simulink model "ER_Simulink"  (R2016b)
settings: Solver=VariableStepAuto  StartTime=0.01  StopTime=10.0  RelTol=1e-3  EnableMultiTasking=on
undefined symbols (not defined in the file or in its folder): sigbuilder_block
settings Model: Creator=Administrator  LastModifiedBy=maelula
settings DataIOCC: LimitDataPoints=on  SaveFormat=Array
settings OptimizationCC: LifeSpan=inf
settings DebuggingCC: SolverPrmCheckMsg=warning  SFUnexpectedBacktrackingDiag=warning  SFNoUnconditionalDefaultTransitionDiag=warning  SFExecutionAtInitializationDiag=none
settings HardwareCC: ProdBitPerPointer=32  ProdBitPerSizeT=32  ProdBitPerPtrDiffT=32  ProdLargestAtomicFloat=None  ProdIntDivRoundTo=Undefined  ProdEndianess=Unspecified  ProdWordSize=32  ProdHWDeviceType=32-bit Generic
settings ModelReferenceCC: PropagateSignalLabelsOutOfModel=off
settings GRTTargetCC: TargetLangStandard=C89/C90 (ANSI)  GeneratePreprocessorConditionals=Disable all
settings ConfigComp: CovMetricSettings=dw  CovHtmlReporting=on  CovSaveCumulativeToWorkspaceVar=on  CovSaveSingleToWorkspaceVar=on  CovExternalEMLEnable=off  CovSFcnEnable=off

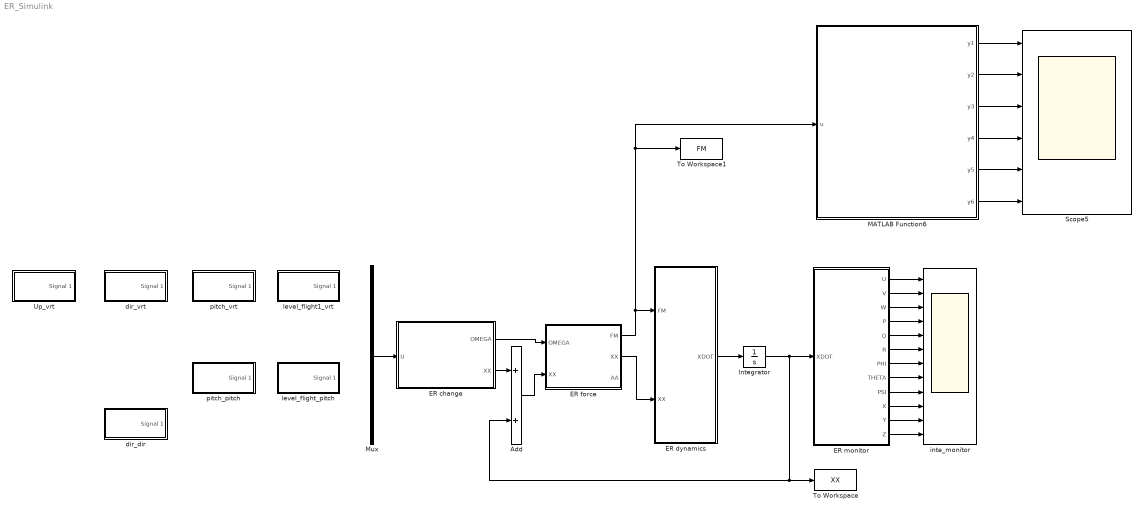
== system ER_Simulink ==
  Add : Sum
  "ER change " : MATLAB Function  TreatAsAtomicUnit=on
  "ER dynamics " : MATLAB Function  TreatAsAtomicUnit=on
  ER force : MATLAB Function  TreatAsAtomicUnit=on
  ER monitor : MATLAB Function  TreatAsAtomicUnit=on
  Integrator : Integrator
  MATLAB Function6 : MATLAB Function  TreatAsAtomicUnit=on
  Mux : Mux
  Scope5 : Scope  NumInputPorts=6
  To Workspace : ToWorkspace  VariableName=XX  SampleTime=-1
  To Workspace1 : ToWorkspace  VariableName=FM  SampleTime=-1
  Up_vrt : Subsystem  Tag=STV Subsys  LoadFcn=sigbuilder_block('load');  StartFcn=sigbuilder_block('start');  StopFcn=sigbuilder_block('stop');  ClipboardFcn=sigbuilder_block('clipboard');  mask(Sigbuilder block){tuvar=[0:10]}
      mask help: Simulink:masks:SigbuilderBlock_MD
      mask init:
      | if ~strcmp(get_param(bdroot(gcbh),'SimulationStatus'),'stopped') tuvar = sigbuilder_block('maskInit'); end
      settings: CopyFcn=sigbuilder_block('copy');  DeleteFcn=sigbuilder_block('delete');  ModelCloseFcn=sigbuilder_block('modelClose');  PreSaveFcn=sigbuilder_block('preSave');  PauseFcn=sigbuilder_block('pause');  ContinueFcn=sigbuilder_block('continue');  NameChangeFcn=sigbuilder_block('namechange');  OpenFcn=sigbuilder_block('open',[327 194 749 530 ]);  CloseFcn=sigbuilder_block('close');
      mask Display: plot(0, 0, 100, 100,[2, 2, 32, 32, 2], [68, 8, 8, 68, 68],[32, 2], [38, 38], [32, 19, 2],[53, 60, 44], [32, 17, 17, 2],[16, 16, 31, 31]);txt = getActiveGroup(gcbh);text(2, 100, txt,'verticalAlignment', 'top');
  dir_dir : Subsystem  Tag=STV Subsys  LoadFcn=sigbuilder_block('load');  StartFcn=sigbuilder_block('start');  StopFcn=sigbuilder_block('stop');  ClipboardFcn=sigbuilder_block('clipboard');  mask(Sigbuilder block){tuvar=[0:10]}
      mask help: Simulink:masks:SigbuilderBlock_MD
      mask init:
      | if ~strcmp(get_param(bdroot(gcbh),'SimulationStatus'),'stopped') tuvar = sigbuilder_block('maskInit'); end
      settings: CopyFcn=sigbuilder_block('copy');  DeleteFcn=sigbuilder_block('delete');  ModelCloseFcn=sigbuilder_block('modelClose');  PreSaveFcn=sigbuilder_block('preSave');  PauseFcn=sigbuilder_block('pause');  ContinueFcn=sigbuilder_block('continue');  NameChangeFcn=sigbuilder_block('namechange');  OpenFcn=sigbuilder_block('open',[304 160 891 552 ]);  CloseFcn=sigbuilder_block('close');
      mask Display: plot(0, 0, 100, 100,[2, 2, 32, 32, 2], [68, 8, 8, 68, 68],[32, 2], [38, 38], [32, 19, 2],[53, 60, 44], [32, 17, 17, 2],[16, 16, 31, 31]);txt = getActiveGroup(gcbh);text(2, 100, txt,'verticalAlignment', 'top');
  dir_vrt : Subsystem  Tag=STV Subsys  LoadFcn=sigbuilder_block('load');  StartFcn=sigbuilder_block('start');  StopFcn=sigbuilder_block('stop');  ClipboardFcn=sigbuilder_block('clipboard');  mask(Sigbuilder block){tuvar=[0:10]}
      mask help: Simulink:masks:SigbuilderBlock_MD
      mask init:
      | if ~strcmp(get_param(bdroot(gcbh),'SimulationStatus'),'stopped') tuvar = sigbuilder_block('maskInit'); end
      settings: CopyFcn=sigbuilder_block('copy');  DeleteFcn=sigbuilder_block('delete');  ModelCloseFcn=sigbuilder_block('modelClose');  PreSaveFcn=sigbuilder_block('preSave');  PauseFcn=sigbuilder_block('pause');  ContinueFcn=sigbuilder_block('continue');  NameChangeFcn=sigbuilder_block('namechange');  OpenFcn=sigbuilder_block('open',[232 176 799 559 ]);  CloseFcn=sigbuilder_block('close');
      mask Display: plot(0, 0, 100, 100,[2, 2, 32, 32, 2], [68, 8, 8, 68, 68],[32, 2], [38, 38], [32, 19, 2],[53, 60, 44], [32, 17, 17, 2],[16, 16, 31, 31]);txt = getActiveGroup(gcbh);text(2, 100, txt,'verticalAlignment', 'top');
  inte_monitor : Scope  NumInputPorts=12
  "level_flight1_vrt " : Subsystem  Tag=STV Subsys  LoadFcn=sigbuilder_block('load');  StartFcn=sigbuilder_block('start');  StopFcn=sigbuilder_block('stop');  ClipboardFcn=sigbuilder_block('clipboard');  mask(Sigbuilder block){tuvar=[0:10]}
      mask help: Simulink:masks:SigbuilderBlock_MD
      mask init:
      | if ~strcmp(get_param(bdroot(gcbh),'SimulationStatus'),'stopped') tuvar = sigbuilder_block('maskInit'); end
      settings: CopyFcn=sigbuilder_block('copy');  DeleteFcn=sigbuilder_block('delete');  ModelCloseFcn=sigbuilder_block('modelClose');  PreSaveFcn=sigbuilder_block('preSave');  PauseFcn=sigbuilder_block('pause');  ContinueFcn=sigbuilder_block('continue');  NameChangeFcn=sigbuilder_block('namechange');  OpenFcn=sigbuilder_block('open',[470 231 709 500 ]);  CloseFcn=sigbuilder_block('close');
      mask Display: plot(0, 0, 100, 100,[2, 2, 32, 32, 2], [68, 8, 8, 68, 68],[32, 2], [38, 38], [32, 19, 2],[53, 60, 44], [32, 17, 17, 2],[16, 16, 31, 31]);txt = getActiveGroup(gcbh);text(2, 100, txt,'verticalAlignment', 'top');
  level_flight_pitch : Subsystem  Tag=STV Subsys  LoadFcn=sigbuilder_block('load');  StartFcn=sigbuilder_block('start');  StopFcn=sigbuilder_block('stop');  ClipboardFcn=sigbuilder_block('clipboard');  mask(Sigbuilder block){tuvar=[0:10]}
      mask help: Simulink:masks:SigbuilderBlock_MD
      mask init:
      | if ~strcmp(get_param(bdroot(gcbh),'SimulationStatus'),'stopped') tuvar = sigbuilder_block('maskInit'); end
      settings: CopyFcn=sigbuilder_block('copy');  DeleteFcn=sigbuilder_block('delete');  ModelCloseFcn=sigbuilder_block('modelClose');  PreSaveFcn=sigbuilder_block('preSave');  PauseFcn=sigbuilder_block('pause');  ContinueFcn=sigbuilder_block('continue');  NameChangeFcn=sigbuilder_block('namechange');  OpenFcn=sigbuilder_block('open',[139 266 709 484 ]);  CloseFcn=sigbuilder_block('close');
      mask Display: plot(0, 0, 100, 100,[2, 2, 32, 32, 2], [68, 8, 8, 68, 68],[32, 2], [38, 38], [32, 19, 2],[53, 60, 44], [32, 17, 17, 2],[16, 16, 31, 31]);txt = getActiveGroup(gcbh);text(2, 100, txt,'verticalAlignment', 'top');
  pitch_pitch : Subsystem  Tag=STV Subsys  LoadFcn=sigbuilder_block('load');  StartFcn=sigbuilder_block('start');  StopFcn=sigbuilder_block('stop');  ClipboardFcn=sigbuilder_block('clipboard');  mask(Sigbuilder block){tuvar=[0:10]}
      mask help: Simulink:masks:SigbuilderBlock_MD
      mask init:
      | if ~strcmp(get_param(bdroot(gcbh),'SimulationStatus'),'stopped') tuvar = sigbuilder_block('maskInit'); end
      settings: CopyFcn=sigbuilder_block('copy');  DeleteFcn=sigbuilder_block('delete');  ModelCloseFcn=sigbuilder_block('modelClose');  PreSaveFcn=sigbuilder_block('preSave');  PauseFcn=sigbuilder_block('pause');  ContinueFcn=sigbuilder_block('continue');  NameChangeFcn=sigbuilder_block('namechange');  OpenFcn=sigbuilder_block('open',[139 266 709 484 ]);  CloseFcn=sigbuilder_block('close');
      mask Display: plot(0, 0, 100, 100,[2, 2, 32, 32, 2], [68, 8, 8, 68, 68],[32, 2], [38, 38], [32, 19, 2],[53, 60, 44], [32, 17, 17, 2],[16, 16, 31, 31]);txt = getActiveGroup(gcbh);text(2, 100, txt,'verticalAlignment', 'top');
  pitch_vrt : Subsystem  Tag=STV Subsys  LoadFcn=sigbuilder_block('load');  StartFcn=sigbuilder_block('start');  StopFcn=sigbuilder_block('stop');  ClipboardFcn=sigbuilder_block('clipboard');  mask(Sigbuilder block){tuvar=[0:10]}
      mask help: Simulink:masks:SigbuilderBlock_MD
      mask init:
      | if ~strcmp(get_param(bdroot(gcbh),'SimulationStatus'),'stopped') tuvar = sigbuilder_block('maskInit'); end
      settings: CopyFcn=sigbuilder_block('copy');  DeleteFcn=sigbuilder_block('delete');  ModelCloseFcn=sigbuilder_block('modelClose');  PreSaveFcn=sigbuilder_block('preSave');  PauseFcn=sigbuilder_block('pause');  ContinueFcn=sigbuilder_block('continue');  NameChangeFcn=sigbuilder_block('namechange');  OpenFcn=sigbuilder_block('open',[232 176 799 559 ]);  CloseFcn=sigbuilder_block('close');
      mask Display: plot(0, 0, 100, 100,[2, 2, 32, 32, 2], [68, 8, 8, 68, 68],[32, 2], [38, 38], [32, 19, 2],[53, 60, 44], [32, 17, 17, 2],[16, 16, 31, 31]);txt = getActiveGroup(gcbh);text(2, 100, txt,'verticalAlignment', 'top');
  wires:
  "ER change "/1(OMEGA) -> ER force/1(OMEGA)
  Mux/1 -> "ER change "/1(U)
  ER monitor/2(V) -> inte_monitor/2
  ER monitor/4(P) -> inte_monitor/4
  ER monitor/5(Q) -> inte_monitor/5
  ER monitor/6(R) -> inte_monitor/6
  ER monitor/8(THETA) -> inte_monitor/8
  ER monitor/11(Y) -> inte_monitor/11
  ER monitor/7(PHI) -> inte_monitor/7
  ER monitor/9(PSI) -> inte_monitor/9
  ER monitor/10(X) -> inte_monitor/10
  "ER dynamics "/1(XDOT) -> Integrator/1
  Add/1 -> ER force/2("XX ")
  ER force/2(XX) -> "ER dynamics "/2(XX)
  MATLAB Function6/1(y1) -> Scope5/1
  MATLAB Function6/2(y2) -> Scope5/2
  MATLAB Function6/4(y4) -> Scope5/4
  MATLAB Function6/5(y5) -> Scope5/5
  MATLAB Function6/6(y6) -> Scope5/6
  ER force/1(FM) -> "ER dynamics "/1(FM), To Workspace1/1, MATLAB Function6/1(u)
  Integrator/1 -> ER monitor/1(XDOT), To Workspace/1, Add/2
  "ER change "/2(XX) -> Add/1
  ER monitor/12(Z) -> inte_monitor/12
  ER monitor/3(W) -> inte_monitor/3
  MATLAB Function6/3(y3) -> Scope5/3
  ER monitor/1(U) -> inte_monitor/1

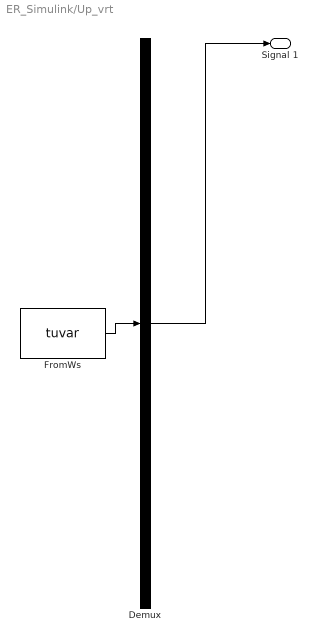
== system ER_Simulink/Up_vrt ==
  Demux : Demux  Tag=STV Demux  Outputs=1
  FromWs : FromWorkspace  Tag=STV FromWs  VariableName=tuvar  SampleTime=0
      SigBuilderData=|
      | common.afterFinalStr = 'Extrapolate'
      | common.sampleTime = 0
      | dataSet.timeRange = [0 10]
      | dataSet.name = 'Group 1'
      | sbobj.Groups.Name = 'Group 1'
      | sbobj.Groups.Signals.Name = 'Signal 1'
      | sbobj.Groups.Signals.XData = [0 3 5 10]
      | sbobj.Groups.Signals.YData = [200 200 167.1876 167.1876]
  Signal 1 : Outport  Tag=STV Outport
  wires:
  Demux/1 -> Signal 1/1
  FromWs/1 -> Demux/1

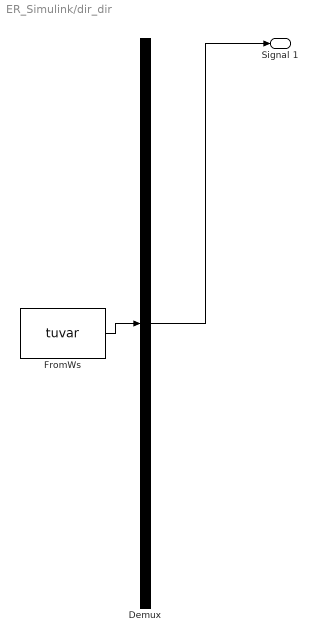
== system ER_Simulink/dir_dir ==
  Demux : Demux  Tag=STV Demux  Outputs=1
  FromWs : FromWorkspace  Tag=STV FromWs  VariableName=tuvar  SampleTime=0
      SigBuilderData=|
      | common.afterFinalStr = 'Extrapolate'
      | common.sampleTime = 0
      | dataSet.timeRange = [0 10]
      | dataSet.name = 'Group 1'
      | sbobj.Groups.Name = 'Group 1'
      | sbobj.Groups.Signals.Name = 'Signal 1'
      | sbobj.Groups.Signals.XData = [0 4 4 4.4 4.4 10]
      | sbobj.Groups.Signals.YData = [0 0 177.97 177.97 0 0]
  Signal 1 : Outport  Tag=STV Outport
  wires:
  Demux/1 -> Signal 1/1
  FromWs/1 -> Demux/1

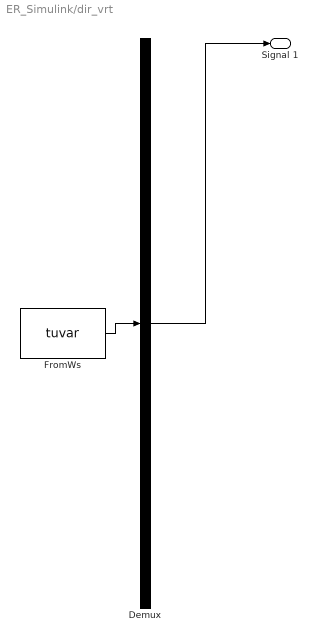
== system ER_Simulink/dir_vrt ==
  Demux : Demux  Tag=STV Demux  Outputs=1
  FromWs : FromWorkspace  Tag=STV FromWs  VariableName=tuvar  SampleTime=0
      SigBuilderData=|
      | common.afterFinalStr = 'Extrapolate'
      | common.sampleTime = 0
      | dataSet.timeRange = [0 10]
      | dataSet.name = 'Group 1'
      | sbobj.Groups.Name = 'Group 1'
      | sbobj.Groups.Signals.Name = 'Signal 1'
      | sbobj.Groups.Signals.XData = [0 1 2 5 7 10]
      | sbobj.Groups.Signals.YData = [200 200 167.188 167.188 167.1876 167.1876]
  Signal 1 : Outport  Tag=STV Outport
  wires:
  Demux/1 -> Signal 1/1
  FromWs/1 -> Demux/1

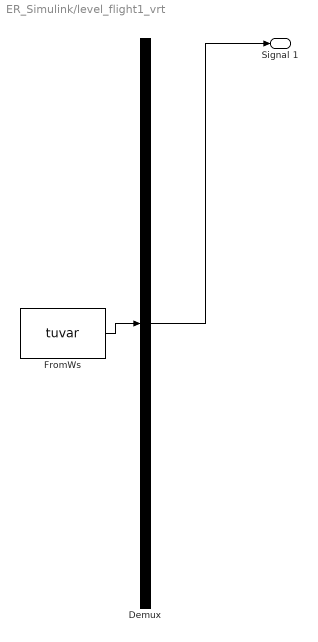
== system ER_Simulink/level_flight1_vrt  ==
  Demux : Demux  Tag=STV Demux  Outputs=1
  FromWs : FromWorkspace  Tag=STV FromWs  VariableName=tuvar  SampleTime=0
      SigBuilderData=|
      | common.afterFinalStr = 'Extrapolate'
      | common.sampleTime = 0
      | dataSet.timeRange = [0 10]
      | dataSet.name = 'Group 1'
      | sbobj.Groups.Name = 'Group 1'
      | sbobj.Groups.Signals.Name = 'Signal 1'
      | sbobj.Groups.Signals.XData = [0 1 4 6 6 10]
      | sbobj.Groups.Signals.YData = [200 200 167.1876 167.1876 198.8207 198.8207]
  Signal 1 : Outport  Tag=STV Outport
  wires:
  Demux/1 -> Signal 1/1
  FromWs/1 -> Demux/1

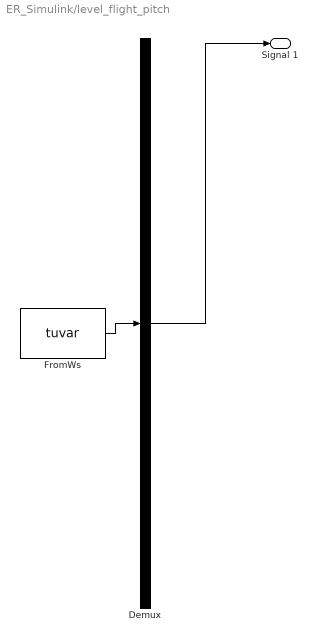
== system ER_Simulink/level_flight_pitch ==
  Demux : Demux  Tag=STV Demux  Outputs=1
  FromWs : FromWorkspace  Tag=STV FromWs  VariableName=tuvar  SampleTime=0
      SigBuilderData=|
      | common.afterFinalStr = 'Extrapolate'
      | common.sampleTime = 0
      | dataSet.timeRange = [0 10]
      | dataSet.name = 'Group 1'
      | sbobj.Groups.Name = 'Group 1'
      | sbobj.Groups.Signals.Name = 'Signal 1'
      | sbobj.Groups.Signals.XData = [0 4 4 4.4 4.4 10]
      | sbobj.Groups.Signals.YData = [0 0 62.895 62.895 0 0]
  Signal 1 : Outport  Tag=STV Outport
  wires:
  Demux/1 -> Signal 1/1
  FromWs/1 -> Demux/1

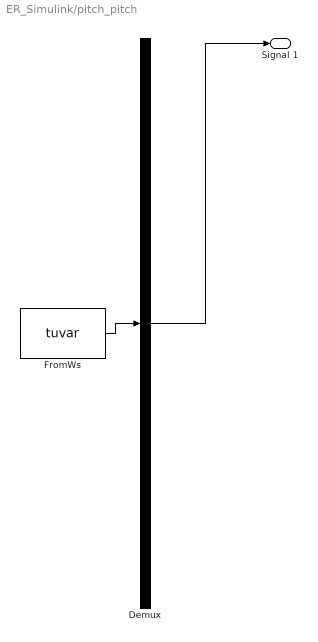
== system ER_Simulink/pitch_pitch ==
  Demux : Demux  Tag=STV Demux  Outputs=1
  FromWs : FromWorkspace  Tag=STV FromWs  VariableName=tuvar  SampleTime=0
      SigBuilderData=|
      | common.afterFinalStr = 'Extrapolate'
      | common.sampleTime = 0
      | dataSet.timeRange = [0 10]
      | dataSet.name = 'Group 1'
      | sbobj.Groups.Name = 'Group 1'
      | sbobj.Groups.Signals.Name = 'Signal 1'
      | sbobj.Groups.Signals.XData = [0 8.6 8.6 9 9 10]
      | sbobj.Groups.Signals.YData = [0 0 62.895 62.895 0 0]
  Signal 1 : Outport  Tag=STV Outport
  wires:
  Demux/1 -> Signal 1/1
  FromWs/1 -> Demux/1

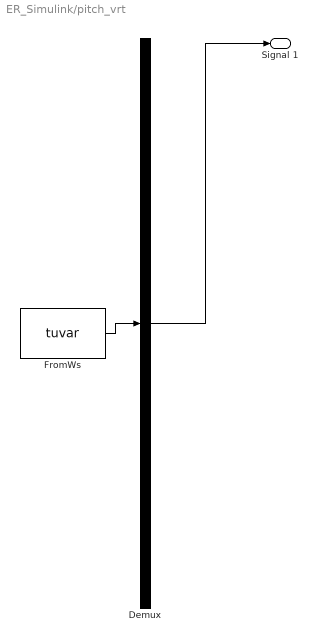
== system ER_Simulink/pitch_vrt ==
  Demux : Demux  Tag=STV Demux  Outputs=1
  FromWs : FromWorkspace  Tag=STV FromWs  VariableName=tuvar  SampleTime=0
      SigBuilderData=|
      | common.afterFinalStr = 'Extrapolate'
      | common.sampleTime = 0
      | dataSet.timeRange = [0 10]
      | dataSet.name = 'Group 1'
      | sbobj.Groups.Name = 'Group 1'
      | sbobj.Groups.Signals.Name = 'Signal 1'
      | sbobj.Groups.Signals.XData = [0 5 7 10]
      | sbobj.Groups.Signals.YData = [200 200 167.188 167.1876]
  Signal 1 : Outport  Tag=STV Outport
  wires:
  Demux/1 -> Signal 1/1
  FromWs/1 -> Demux/1

== matlab function ER_Simulink/ER change  ==
  data: U input; OMEGA output; XX output
function [OMEGA,XX]  =change(U)

%%%%%%%%%%%%%%%%%%%%%%%%%%%%%%%%%%%%%%%%%%%%%%%%
%%%%输入4个转速操纵量
Rvrt = U(1);
Rroll = U(2);
Rpitch = U(3);
Rdir = U(4);

a1=Rvrt*Rvrt;
a2=Rroll*Rroll;
a3=Rpitch*Rpitch;
a4=Rdir*Rdir;

%%%%%%%%%%%%%%%%%%%%%%%%%%%%%%%%%%%%%%%%%%%%%%%%
%%%%将转速操纵量转化为每个螺旋桨的转速
R1=a1+a2+a3-a4;
R2=a1-a2+a3+a4;
R3=a1-a2-a3-a4;
R4=a1+a2-a3+a4;
R5=a1+a2+a3+a4;
R6=a1-a2+a3-a4;
R7=a1-a2-a3+a4;
R8=a1+a2-a3-a4;


OMEGA = [R1;R2;R3;R4;R5;R6;R7;R8];

%%%%%%%%%%%%%%%%%%%%%%%%%%%%%%%%%%%%%%%%%%%%%%%%
%%%%赋予运动学量初值
XX = [0;0;0;0;0;0;0;0;0;0;0;0];

== matlab function ER_Simulink/ER dynamics  ==
  data: FM input; XX input; XDOT output
function XDOT =dynamics(FM,XX)

U = XX(1);
V = XX(2);
W = XX(3);
P = XX(4);
Q = XX(5);
R = XX(6);
PHI = XX(7);
THETA = XX(8);
PSI = XX(9);

FX = FM(1);
FY = FM(2);
FZ = FM(3);
MX = FM(4);
MY = FM(5);
MZ = FM(6);

m = 1.6;

IX = 0.0081;
IY = 0.0081;
IZ = 0.00142;

IZX = 0;

L = MX;
M = MY;
N = MZ;

%%%%%%%%%%%%%%%%%%%%%%%%%%%%%%%%%%%%%%%%%%%%%%%%
%%%%运动学方程解算
Ut = V*R-W*Q+FX/m;
Vt = -U*R+W*P+FY/m;
Wt = U*Q-V*P+FZ/m;

Pt = 1/(IX*IZ-IZX^2)*(IZ*L+IZX*N+IZX*(IX-IY+IZ)*P*Q+(IY*IZ-IZX^2-IZ^2)*Q*R);
Qt = 1/(IY)*(M-(IX-IZ)*P*R-IZX*(P^2-R^2));
Rt = 1/(IX*IZ-IZX^2)*(IZX*L+IX*N+(IX^2-IX*IY+IZX^2)*P*Q-IZX*(IX-IY-IZ)*Q*R);

PHIt = P+tan(THETA)*(Q*sin(PHI)+R*cos(PHI));
THETAt = Q*cos(PHI)-R*sin(PHI);
PSIt = 1/cos(PHI)*(Q*sin(PHI)+R*cos(PHI));

Xt = U*cos(THETA)*cos(PSI)+V*(sin(THETA)*sin(PHI)*cos(PSI)-cos(PHI)*sin(PSI))+W*(sin(THETA)*cos(PHI)*cos(PSI)+sin(PHI)*sin(PSI));
Yt = U*cos(THETA)*sin(PSI)+V*(sin(THETA)*sin(PHI)*sin(PSI)+cos(PHI)*cos(PSI))+W*(sin(THETA)*cos(PHI)*sin(PSI)-sin(PHI)*cos(PSI));
Zt = -U*sin(THETA)+V*sin(PHI)*cos(THETA)+W*cos(PHI)*cos(THETA);

XDOT = [Ut;Vt;Wt;Pt;Qt;Rt;PHIt;THETAt;PSIt;Xt;Yt;Zt];

== matlab function ER_Simulink/ER monitor ==
  data: XDOT input; U output; V output; W output; P output; Q output; R output; PHI output; THETA output; PSI output; X output; Y output; Z output
function [U,V,W,P,Q,R,PHI,THETA,PSI,X,Y,Z] = monitor(XDOT)

% y1 = XDOT(1);
% y2 = XDOT(1);
% y3 = XDOT(1);
% y4 = XDOT(1);
% y5 = XDOT(1);
% y6 = XDOT(1);
% y7 = XDOT(1);
% y8 = XDOT(1);
% y9 = XDOT(1);
% y10 = XDOT(1);
% y11 = XDOT(1);
% y12 = XDOT(1);

U = -XDOT(1);
V = -XDOT(2);
W = -XDOT(3);
P = XDOT(4);
Q = XDOT(5);
R = XDOT(6);
PHI = XDOT(7);
THETA = XDOT(8);
PSI = XDOT(9);
X = -XDOT(10);
Y = -XDOT(11);
Z = -XDOT(12);

== matlab function ER_Simulink/ER force ==
  data: OMEGA input; XX input; FM output; XX output; AA output
function [FM,XX,AA]=force(OMEGA,XX)

Fx1=0;
Fy1=0;
l=0.5;
ll=sqrt(2);
rou=1.225;
k1=5.73*10^(-5);
k2=2.53*10^(-6);

OMEGA1S=OMEGA(1);
OMEGA2S=OMEGA(2);
OMEGA3S=OMEGA(3);
OMEGA4S=OMEGA(4);
OMEGA5S=OMEGA(5);
OMEGA6S=OMEGA(6);
OMEGA7S=OMEGA(7);
OMEGA8S=OMEGA(8);

%%%%%%%%%%%%%%%%%%%%%%%%%%%%%%%%%%%%%%%%%%%%%%%%
%%%%计算机体轴系上操纵量引起的力和力矩
L1=rou*k1*OMEGA1S;
L2=rou*k1*OMEGA2S;
L3=rou*k1*OMEGA3S;
L4=rou*k1*OMEGA4S;
L5=rou*k1*OMEGA5S;
L6=rou*k1*OMEGA6S;
L7=rou*k1*OMEGA7S;
L8=rou*k1*OMEGA8S;

Fz1=-(L1+L2+L3+L4+L5+L6+L7+L8);
Mx1=1/ll*l*(L1-L2-L3+L4+L5-L6-L7+L8);
My1=1/ll*l*(L1+L2-L3-L4+L5+L6-L7-L8);
Mz1=k2/k1*(-L1+L2-L3+L4+L5-L6+L7-L8);

%%%%%%%%%%%%%%%%%%%%%%%%%%%%%%%%%%%%%%%%%%%%%%%%
%%%%计算气动力：从气流轴系转换到机体轴系
CD=0.8;
u=XX(1,1);
v=XX(2,1);
w=XX(3,1);
V=(u^2+v^2+w^2)^0.5;

Ax=-CD*V*u;
Ay=-CD*V*v;
Az=-CD*V*w;

%%%%%%%%%%%%%%%%%%%%%%%%%%%%%%%%%%%%%%%%%%%%%%%%
%%%%解算重力：从地面轴系转换到机体轴系
m = 1.6;
g = 9.81;

PHI = XX(7,1);
THETA = XX(8,1);
PSI = XX(9,1);

Lx = [cos(PHI) sin(PHI) 0;
      -sin(PHI) cos(PHI) 0;
      0 0 1];
Ly = [cos(THETA) 0 -sin(THETA);
      0 1 0;
      sin(THETA) 0 cos(THETA)];
Lz = [1 0 0;
      0 cos(PSI) sin(PSI);
      0 -sin(PSI) cos(PSI)];

DCM = Lx*Ly*Lz;
gforce = DCM*[0,0,m*g]';

%%%%%%%%%%%%%%%%%%%%%%%%%%%%%%%%%%%%%%%%%%%%%%%%
%%%%粗略计算机体轴系上阻尼力矩
p=XX(4,1);
q=XX(5,1);
r=XX(6,1);

AMx=-CD*0.5*p;
AMy=-CD*0.5*q;
AMz=-CD*0.5*r;

% AMx=0;
% AMy=0;
% AMz=0;

%%%%%%%%%%%%%%%%%%%%%%%%%%%%%%%%%%%%%%%%%%%%%%%%
%%%%计算输出：
%%%%机体轴系三方向受力=操纵力+气动力+重力：
Fx=Fx1+Ax+gforce(1);
Fy=Fy1+Ay+gforce(2);
Fz=Fz1+Az+gforce(3);

%%%%%%%%%%%%%%%%%%%%%%%%%%%%%%%%%%%%%%%%%%%%%%%%
%%%%机体轴系三方向力矩=操纵力矩+阻尼力矩：
Mx=Mx1+AMx;
My=My1+AMy;
Mz=Mz1+AMz;

FM=[Fx;Fy;Fz;Mx;My;Mz];
AA=[Ax;Ay;Az];

== matlab function ER_Simulink/MATLAB Function6 ==
  data: u input; y1 output; y2 output; y3 output; y4 output; y5 output; y6 output
function [y1,y2,y3,y4,y5,y6] = fcn(u)

y1 = u(1);
y2 = u(2);
y3 = u(3);
y4 = u(4);
y5 = u(5);
y6 = u(6);
